simulink model "window_in_window_out_fixed"  (R2019b)
settings: Solver=VariableStepAuto  StartTime=0.0  StopTime=7  RelTol=1e-3
undefined symbols (not defined in the file): xc7vx485tffg1157
libraries: ModelComposer x5
settings Model: Creator=viswanad  LastModifiedBy=abehbood
settings DataIOCC: ReturnWorkspaceOutputs=off
settings SFSimCC: CustomCodeUndefinedFunction=UseInterfaceOnly

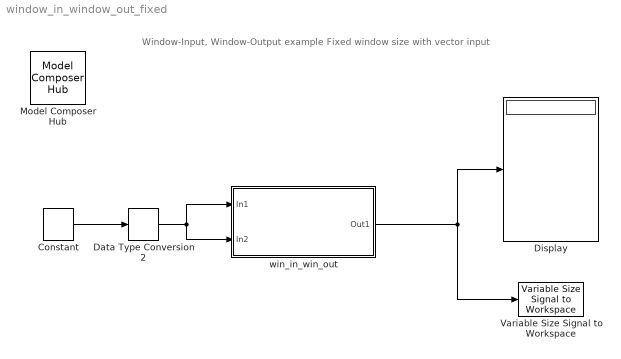
== system window_in_window_out_fixed ==
  note: Window-Input, Window-Output example
      | Fixed window size with vector input
  Constant : ModelComposer/Constant  Value=[1 2 3 4 5 6 7 8 1 2 3 4 5 6 7 8]  SampleTime=1  OutDataType=double  TypeExp=''  Signedness=Signed  WordLength=16  FractionalLength=0  RoundingMode=Truncation to minus infinity  OverflowMode=Wrap around
  Data Type Conversion2 : ModelComposer/Data Type Conversion  OutDataType=int16  TypeExp=''  Signedness=Signed  WordLength=16  FractionalLength=0  RoundingMode=Truncation to minus infinity  OverflowMode=Wrap around
  Display : Display
  Model Composer Hub : ModelComposer/Model Composer Hub  CodeGeneration=off  SubsystemName=win_in_win_out  TargetDirectory=./code  ExportType=AI Engines  IpVendor=xilinx.com  IpLibrary=hls  IpVersion=1.0  IpHWLanguage=Verilog  AieCompilerOptions={}  CreateTestbench=on  TestbenchStackSize=10  RunAieSim=off  AieSimTimeout=50000  LaunchVitisAnalyzer=off  RunX86Sim=off  X86SimTimeout=10  ProjDevice=xc7vx485tffg1157-1  ProjDevicePart=xc7vx485tffg1157-1  SamplePeriod=-1  ClockFrequency=200  DataPathParallelism=1
  Variable Size Signal to Workspace : ModelComposer/Variable Size Signal to Workspace  VariableNameMask=simout
  win_in_win_out : Subsystem
  wires:
  win_in_win_out/1(Out1) -> Variable Size Signal to Workspace/1, Display/1
  Data Type Conversion2/1 -> win_in_win_out/1(In1), win_in_win_out/2(In2)
  Constant/1 -> Data Type Conversion2/1

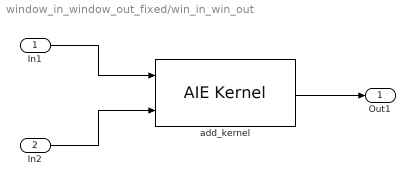
== system window_in_window_out_fixed/win_in_win_out ==
  In1 : Inport
  In2 : Inport  Port=2
  add_kernel : ModelComposer/AIE Kernel  PortAttributesTable={ 'Input', 'inw1', 'input_window_int16 *', '16', '0', 'sync', ''; 'Input', 'inw2', 'input_window_int16 *', '16', '0', 'sync', ''; 'Output', 'outw', 'output_window_int16 *', '16', '', 'sync', '' }  PortAttributesEnablement={'off', 'off', 'off', 'on', 'on', 'on', 'off';'off', 'off', 'off', 'on', 'on', 'on', 'off';'off', 'off', 'off', 'on', 'off', 'on', 'off'}  FormalArgDecls={'input_window_int16 * inw1', 'input_window_int16 * inw2', 'output_window_int16 * outw'}  PortWindowSizes={1.600000000000000000e+01; 1.600000000000000000e+01; 1.600000000000000000e+01}  PortWindowMargins={0.000000000000000000e+00; 0.000000000000000000e+00; 0.000000000000000000e+00}  PortSynchronicities={'sync'; 'sync'; 'sync'}  PortSignalSizes={0.000000000000000000e+00; 0.000000000000000000e+00; 0.000000000000000000e+00}  SimLibPath=''  FunctionTabVisible=on  FunctionDescription=void add_kernel(input_window_int16 * inw1, input_window_int16 * inw2, output_window_int16 * outw)  KernelHeaderFile=src/kernels/window_in_window_out_fixed_size.h  KernelFunction=add_kernel  KernelFunctionSelect=<empty>  KernelSourceFile=src/kernels/window_in_window_out_fixed_size.cc  KernelSearchPaths={}  PreProcOptions={}  CoreRuntimeRatio=0.9  KernelLocSpec=off  ColRowLocation=[0 0]
  Out1 : Outport  VectorParamsAs1DForOutWhenUnconnected=off
  wires:
  In1/1 -> add_kernel/1
  add_kernel/1 -> Out1/1
  In2/1 -> add_kernel/2
